simulink model "test"  (R2018b)
settings: Solver=VariableStepAuto  StartTime=0.0  StopTime=10.0  RelTol=1e-3
undefined symbols (not defined in the file or in its folder): Den, Kden, KNum, Num, Pden, PNum
settings Model: Creator=57531  LastModifiedBy=57531

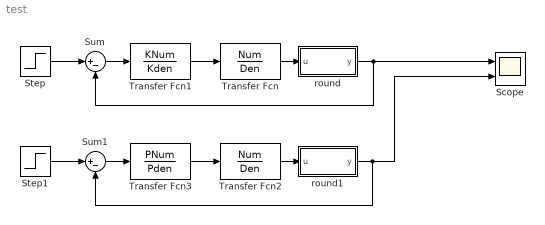
== system test ==
  Scope : Scope  NumInputPorts=2
  Step : Step  SampleTime=0
  Step1 : Step  SampleTime=0
  Sum : Sum  Inputs=|+-
  Sum1 : Sum  Inputs=|+-
  Transfer Fcn : TransferFcn  Numerator=Num  Denominator=Den
  Transfer Fcn1 : TransferFcn  Numerator=KNum  Denominator=Kden
  Transfer Fcn2 : TransferFcn  Numerator=Num  Denominator=Den
  Transfer Fcn3 : TransferFcn  Numerator=PNum  Denominator=Pden
  round : MATLAB Function  TreatAsAtomicUnit=on
  round1 : MATLAB Function  TreatAsAtomicUnit=on
  wires:
  Transfer Fcn1/1 -> Transfer Fcn/1
  Sum/1 -> Transfer Fcn1/1
  Sum1/1 -> Transfer Fcn3/1
  Transfer Fcn3/1 -> Transfer Fcn2/1
  Transfer Fcn/1 -> round/1(u)
  Transfer Fcn2/1 -> round1/1(u)
  Step/1 -> Sum/1
  Step1/1 -> Sum1/1
  round/1(y) -> Scope/1, Sum/2
  round1/1(y) -> Scope/2, Sum1/2

== matlab function test/round1 ==
  data: u input; y output
function y = fcn(u)
y = round(u * 10000) / 10000;

== matlab function test/round ==
  data: u input; y output
function y = fcn(u)
y = round(u * 50000) / 50000;
